simulink model "Motor_Model_sim"  (R2022b)
settings: Solver=ode1be  StartTime=0.0  StopTime=10.0  FixedStep=1e-3  RelTol=1e-3
undefined symbols (not defined in the file or in its folder): motor
settings Model: Creator=gotta  LastModifiedBy=gotta

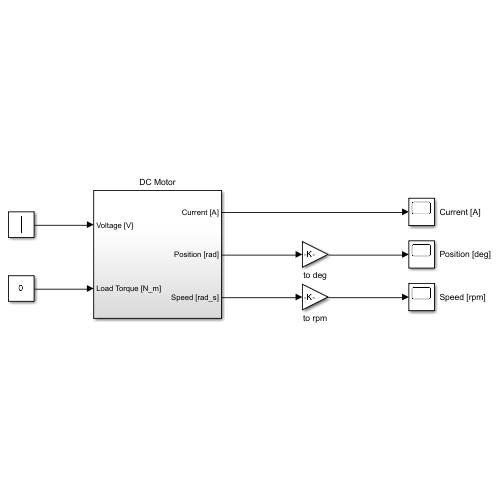
[thumbnail: Simulink's stored preview of the top-level diagram]
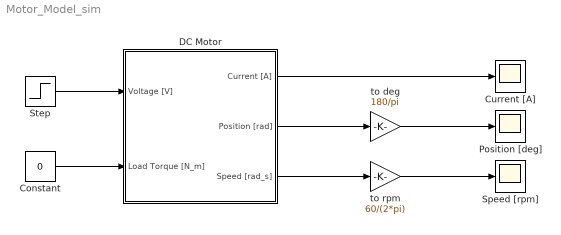
== system Motor_Model_sim ==
  Constant : Constant  Value=0
  Current [A] : Scope
  DC Motor : Subsystem
  Position [deg] : Scope
  Speed [rpm] : Scope
  Step : Step  After=5  SampleTime=0
  to deg : Gain  Gain=180/pi
  to rpm : Gain  Gain=60/(2*pi)
  wires:
  Constant/1 -> DC Motor/2(Load Torque [N_m])
  Step/1 -> DC Motor/1(Voltage [V])
  DC Motor/2(Position [rad]) -> to deg/1
  to deg/1 -> Position [deg]/1
  to rpm/1 -> Speed [rpm]/1
  DC Motor/3(Speed [rad_s]) -> to rpm/1
  DC Motor/1(Current [A]) -> Current [A]/1

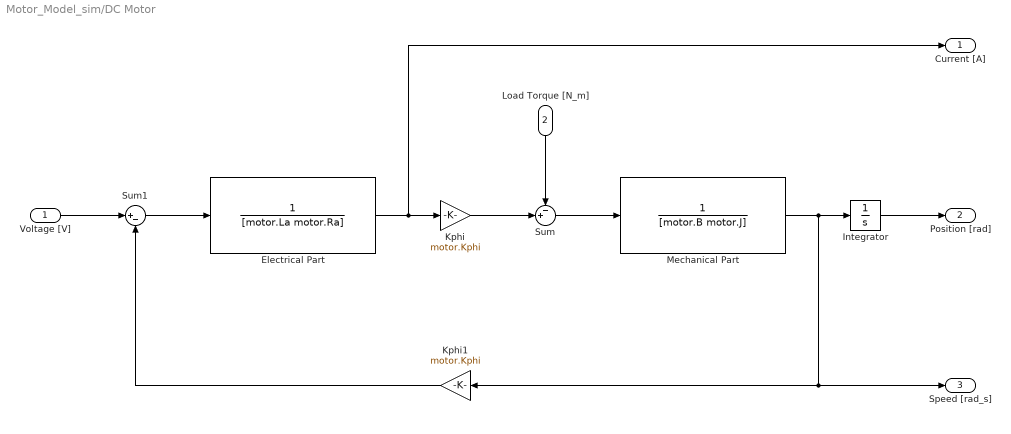
== system Motor_Model_sim/DC Motor ==
  Voltage [V] : Inport
  Load Torque [N_m] : Inport  Port=2
  Electrical Part : TransferFcn  Denominator=[motor.La motor.Ra]
  Integrator : Integrator
  Kphi : Gain  Gain=motor.Kphi
  Kphi1 : Gain  Gain=motor.Kphi
  Mechanical Part : TransferFcn  Denominator=[motor.B motor.J]
  Sum : Sum  Inputs=-+|
  Sum1 : Sum  Inputs=|+-
  Current [A] : Outport
  Position [rad] : Outport  Port=2
  Speed [rad_s] : Outport  Port=3
  wires:
  Mechanical Part/1 -> Integrator/1, Kphi1/1, Speed [rad_s]/1
  Kphi1/1 -> Sum1/2
  Voltage [V]/1 -> Sum1/1
  Sum1/1 -> Electrical Part/1
  Load Torque [N_m]/1 -> Sum/1
  Kphi/1 -> Sum/2
  Electrical Part/1 -> Current [A]/1, Kphi/1
  Sum/1 -> Mechanical Part/1
  Integrator/1 -> Position [rad]/1
